simulink model "Project1part2_abhaykela"  (R2014b)
settings: Solver=ode5  StartTime=0.0  StopTime=tf0  FixedStep=0.01  RelTol=1e-3
values from neighbouring files (symbols this model uses):
  x0 = [4;-4]    [HW3_Countorplot.m]    (also in HW3_DFPM_AbhayKela.m = [x01;x02]; HW3_NewtonMethod_AbhayKela.m; HW3_PowellsMethod_AbhayKela.m; Project1_AbhayKela_Combined.m = -4.2)
  xdot0 = 10    [Project1_AbhayKela_Combined.m]
settings Model: Creator=axk7578  LastModifiedBy=axk7578

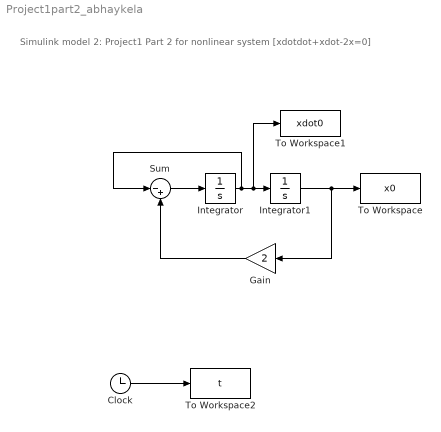
== system Project1part2_abhaykela ==
  note: Simulink model 2: Project1 Part 2 for nonlinear system [xdotdot+xdot-2x=0]
  Clock : Clock
  Gain : Gain  Gain=2
  Integrator : Integrator  InitialCondition=xdot0
  Integrator1 : Integrator  InitialCondition=x0
  Sum : Sum  Inputs=|-+
  To Workspace : ToWorkspace  VariableName=x0  SampleTime=-1
  To Workspace1 : ToWorkspace  VariableName=xdot0  SampleTime=-1
  To Workspace2 : ToWorkspace  VariableName=t  SampleTime=-1
  wires:
  Integrator1/1 -> Gain/1, To Workspace/1
  Sum/1 -> Integrator/1
  Clock/1 -> To Workspace2/1
  Gain/1 -> Sum/2
  Integrator/1 -> Sum/1, To Workspace1/1, Integrator1/1
